simulink model "inv_Pendulum"  (R2017a)
settings: Solver=VariableStepAuto  StartTime=0.0  StopTime=50  RelTol=1e-3
undefined symbols (not defined in the file or in its folder): sigbuilder_block
libraries: simulink x1
settings Model: Creator=Utente  LastModifiedBy=Utente

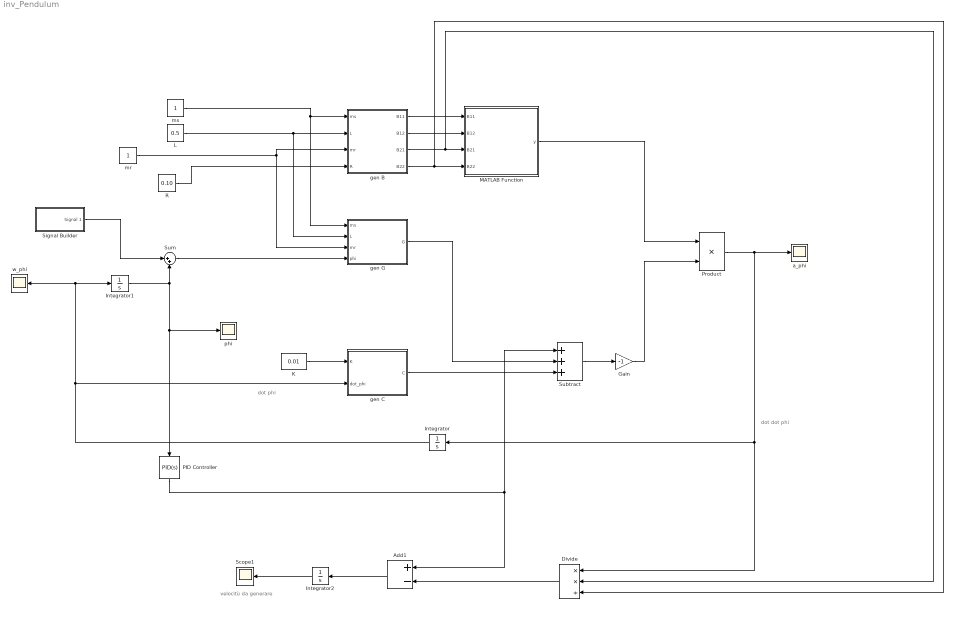
== system inv_Pendulum ==
  note: velocitù da generare
  note: dot dot phi
  note: dot phi
  Add1 : Sum  Inputs=+-
  Divide : Product  Inputs=**/
  Gain : Gain  Gain=-1
  Integrator : Integrator
  Integrator1 : Integrator
  Integrator2 : Integrator
  K : Constant  Value=0.01
  L : Constant  Value=0.5
  MATLAB Function : MATLAB Function  TreatAsAtomicUnit=on
  PID Controller : simulink/Continuous/PID Controller  Controller=PID  TimeDomain=Continuous-time  SampleTime=-1  IntegratorMethod=Forward Euler  FilterMethod=Forward Euler  Form=Parallel  UseFilter=on  ControllerParametersSource=internal  P=565.260311792191  I=2525.8911040342  D=31.061730891796  N=520.590122575615  InitialConditionSource=internal  InitialConditionForIntegrator=0  InitialConditionForFilter=0  ExternalReset=none  LimitOutput=off  UpperSaturationLimit=inf  LowerSaturationLimit=-inf  LinearizeAsGain=on  AntiWindupMode=none  Kb=1  TrackingMode=off  Kt=1  PParamMin=[]  PParamMax=[]  IParamMin=[]  IParamMax=[]  DParamMin=[]  DParamMax=[]  NParamMin=[]  NParamMax=[]  KbParamMin=[]  KbParamMax=[]  KtParamMin=[]  KtParamMax=[]  POutMin=[]  POutMax=[]  IOutMin=[]  IOutMax=[]  DOutMin=[]  DOutMax=[]  NOutMin=[]  NOutMax=[]  KbOutMin=[]  KbOutMax=[]  KtOutMin=[]  KtOutMax=[]  IntegratorOutMin=[]  IntegratorOutMax=[]  FilterOutMin=[]  FilterOutMax=[]  SumOutMin=[]  SumOutMax=[]  SumI1OutMin=[]  SumI1OutMax=[]  SumI2OutMin=[]  SumI2OutMax=[]  SumI3OutMin=[]  SumI3OutMax=[]  SumDOutMin=[]  SumDOutMax=[]  SaturationOutMin=[]  SaturationOutMax=[]  IntegratorContinuousStateAttributes=''  IntegratorStateMustResolveToSignalObject=off  IntegratorRTWStateStorageClass=Auto  FilterContinuousStateAttributes=''  FilterStateMustResolveToSignalObject=off  FilterRTWStateStorageClass=Auto  DifferentiatorICPrevScaledInput=0  DifferentiatorOutMin=[]  DifferentiatorOutMax=[]  InitialConditionSetting=State (most efficient)
  Product : Product
  R : Constant  Value=0.10
  Scope1 : Scope
  Signal Builder : Subsystem  Tag=STV Subsys  LoadFcn=sigbuilder_block('load');  StartFcn=sigbuilder_block('start');  StopFcn=sigbuilder_block('stop');  ClipboardFcn=sigbuilder_block('clipboard');  mask(Sigbuilder block){tuvar=[0:10]}
      mask help: Simulink:masks:SigbuilderBlock_MD
      mask init:
      | if ~strcmp(get_param(bdroot(gcbh),'SimulationStatus'),'stopped') tuvar = sigbuilder_block('maskInit'); end
      settings: CopyFcn=sigbuilder_block('copy');  DeleteFcn=sigbuilder_block('delete');  ModelCloseFcn=sigbuilder_block('modelClose');  PreSaveFcn=sigbuilder_block('preSave');  PauseFcn=sigbuilder_block('pause');  ContinueFcn=sigbuilder_block('continue');  NameChangeFcn=sigbuilder_block('namechange');  OpenFcn=sigbuilder_block('open',[437.6 199.2 550.4 400 ]);  CloseFcn=sigbuilder_block('close');
      mask Display: plot(0, 0, 100, 100,[2, 2, 32, 32, 2], [68, 8, 8, 68, 68],[32, 2], [38, 38], [32, 19, 2],[53, 60, 44], [32, 17, 17, 2],[16, 16, 31, 31]);txt = getActiveGroup(gcbh);text(2, 100, txt,'verticalAlignment', 'top');
  Subtract : Sum  Inputs=+++
  Sum : Sum  Inputs=|++
  a_phi : Scope
  gen B : MATLAB Function  TreatAsAtomicUnit=on
  gen C : MATLAB Function  TreatAsAtomicUnit=on
  "gen G " : MATLAB Function  TreatAsAtomicUnit=on
  mr : Constant
  ms : Constant
  phi : Scope
  w_phi : Scope
  wires:
  Integrator/1 -> Integrator1/1, w_phi/1, gen C/2(dot_phi)
  Product/1 -> Divide/1, Integrator/1, a_phi/1
  Subtract/1 -> Gain/1
  gen B/3(B21) -> Divide/2, MATLAB Function/3(B21)
  mr/1 -> gen B/3(mr), "gen G "/3(mr)
  K/1 -> gen C/1(K)
  ms/1 -> gen B/1(ms), "gen G "/1(ms)
  gen B/1(B11) -> MATLAB Function/1(B11)
  R/1 -> gen B/4(R)
  L/1 -> gen B/2(L), "gen G "/2(L)
  gen B/2(B12) -> MATLAB Function/2(B12)
  "gen G "/1(G) -> Subtract/2
  gen C/1(C) -> Subtract/3
  MATLAB Function/1(y) -> Product/1
  Gain/1 -> Product/2
  Integrator1/1 -> Sum/2, phi/1, PID Controller/1
  PID Controller/1 -> Add1/1, Subtract/1
  Sum/1 -> "gen G "/4(phi)
  Signal Builder/1(Signal 1) -> Sum/1
  Divide/1 -> Add1/2
  gen B/4(B22) -> Divide/3, MATLAB Function/4(B22)
  Add1/1 -> Integrator2/1
  Integrator2/1 -> Scope1/1

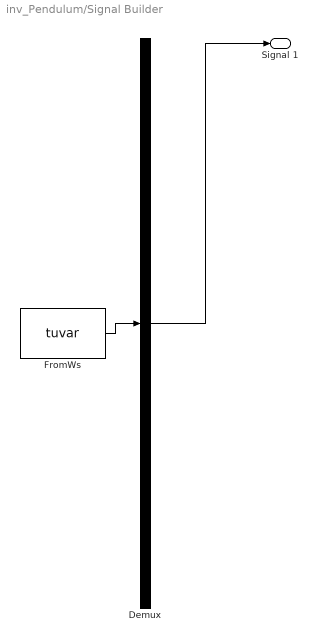
== system inv_Pendulum/Signal Builder ==
  Demux : Demux  Tag=STV Demux  Outputs=1
  FromWs : FromWorkspace  Tag=STV FromWs  VariableName=tuvar  SampleTime=0
      SigBuilderData=|
      | common.afterFinalStr = 'Extrapolate'
      | common.sampleTime = 0
      | dataSet.timeRange = [0 10]
      | dataSet.name = 'Group 1'
      | sbobj.Groups.Name = 'Group 1'
      | sbobj.Groups.Signals.Name = 'Signal 1'
      | sbobj.Groups.Signals.XData = [0 1.02 1.08 1.1 1.1 1.2 1.2 10]
      | sbobj.Groups.Signals.YData = [0 0 0.495 0.505 0.528 0.022 0 0]
  Signal 1 : Outport  Tag=STV Outport
  wires:
  Demux/1 -> Signal 1/1
  FromWs/1 -> Demux/1

== matlab function inv_Pendulum/gen G  ==
  data: ms input; L input; mr input; phi input; G output
function G = fcn(ms,L,mr,phi)
    g = 9.81;
    G = (-ms*g*L/2-mr*g*L)*sin(phi);
end

== matlab function inv_Pendulum/gen B ==
  data: ms input; B11 output; L input; mr input; R input; B12 output; B21 output; B22 output
function [B11,B12,B21,B22] = fcn(ms,L,mr,R)
    g = 9.81; %gravità generica, non localizzata, servirebbe farlo [m/s^2]

    B11 = 0.25*ms*L*L+mr*L*L+0.0833*ms*L*L+mr*R*R;
    B12 = -mr*R*R;
    B21 = -mr*R*R;
    B22 =  mr*R*R;

end

== matlab function inv_Pendulum/gen C ==
  data: K input; dot_phi input; C output
function C = fcn(K,dot_phi)

    C = -K*dot_phi;    
end

== matlab function inv_Pendulum/MATLAB Function ==
  data: B11 input; y output; B12 input; B21 input; B22 input
function y = fcn(B11,B12,B21,B22)

y = 1/(B11-B12*B21/B22);
